simulink model "powersystem"  (R2024a)
settings: Solver=VariableStepAuto  StartTime=0.0  StopTime=10.0  RelTol=1e-3
libraries: spsThreePhaseVIMeasurementLib x6, spsThreePhaseBreakerLib x6, spsThreePhaseTransformerTwoWindingsLib x5, spsRMSLib x4, spsThreePhaseSourceLib x3, spsThreePhaseParallelRLCBranchLib x2, sps_lib x1
settings Model: Creator=acer  LastModifiedBy=acer

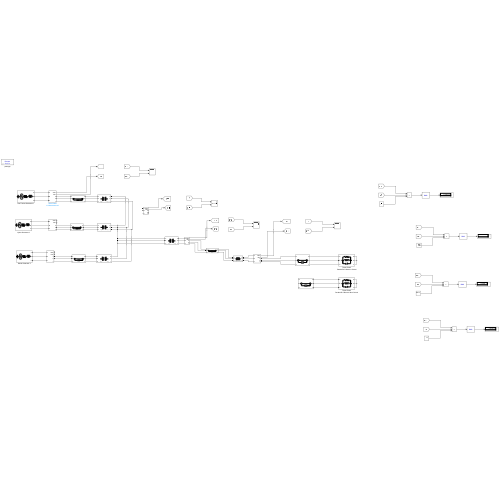
[thumbnail: Simulink's stored preview of the top-level diagram]
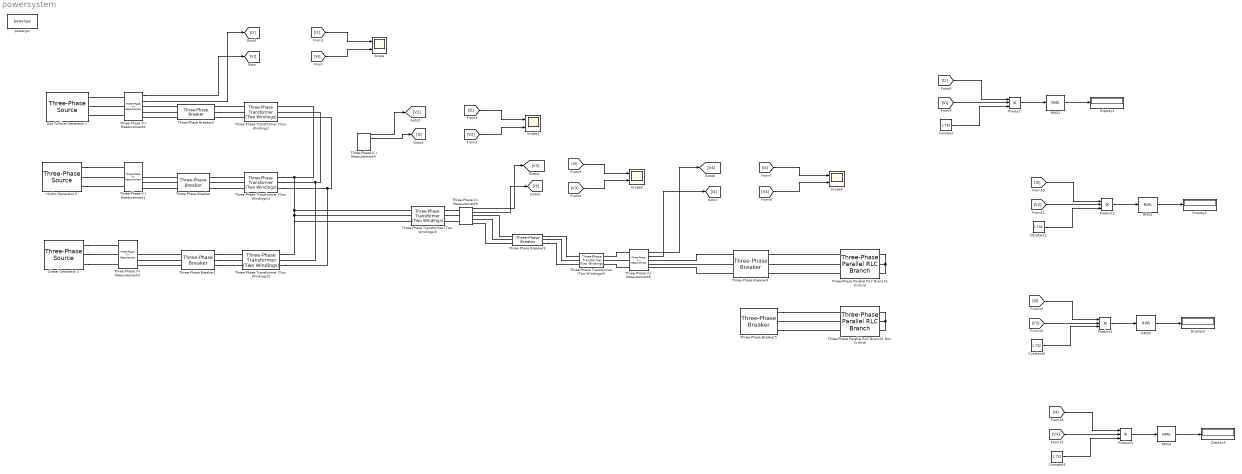
== system powersystem ==
  Constant{,1..3} (4 alike) : Constant  Value=1.732
  Diesel Genarator 3 : spsThreePhaseSourceLib/Three-Phase Source  InternalConnection=Yg  VoltagePhases=off  Voltage=10e3  PhaseAngle=0  Voltage_phases=[25e3 25e3 25e3]/sqrt(3)  PhaseAngles_phases=[0 -120 +120]  Frequency=50  NonIdealSource=on  SpecifyImpedance=off  Resistance=0.8  Inductance=16.58e-3  ShortCircuitLevel=100e6  BaseVoltage=11e3  XRratio=7  BusType=PV  Pref=400e4  Qref=0  Prefabc=[10e3, 10e3, 10e3]  Qrefabc=[0, 0, 0]  Qmin=-inf  Qmax=inf
  Display{1..4} (4 alike) : Display
  Gas Turbine Genarator 1 : spsThreePhaseSourceLib/Three-Phase Source  InternalConnection=Yg  VoltagePhases=off  Voltage=7e3  PhaseAngle=0  Voltage_phases=[25e3 25e3 25e3]/sqrt(3)  PhaseAngles_phases=[0 -120 +120]  Frequency=50  NonIdealSource=on  SpecifyImpedance=off  Resistance=0.8  Inductance=16.58e-3  ShortCircuitLevel=100e6  BaseVoltage=11e3  XRratio=7  BusType=PV  Pref=100e4  Qref=0  Prefabc=[10e3, 10e3, 10e3]  Qrefabc=[0, 0, 0]  Qmin=-inf  Qmax=inf
  Hydro Genarator 2 : spsThreePhaseSourceLib/Three-Phase Source  InternalConnection=Yg  VoltagePhases=off  Voltage=12e3  PhaseAngle=0  Voltage_phases=[25e3 25e3 25e3]/sqrt(3)  PhaseAngles_phases=[0 -120 +120]  Frequency=50  NonIdealSource=on  SpecifyImpedance=off  Resistance=0.8  Inductance=16.58e-3  ShortCircuitLevel=100e6  BaseVoltage=11e3  XRratio=7  BusType=PV  Pref=200e4  Qref=0  Prefabc=[10e3, 10e3, 10e3]  Qrefabc=[0, 0, 0]  Qmin=-inf  Qmax=inf
  Product{,1..3} (4 alike) : Product  Inputs=3
  RMS{1..4} (4 alike) : spsRMSLib/RMS  TrueRMS=on  Freq=60  RMSInit=120  Ts=0
  Scope{,1..3} (4 alike) : Scope  NumInputPorts=2
  Three-Phase Parallel RLC Branch1 Critical : spsThreePhaseParallelRLCBranchLib/Three-Phase Parallel RLC Branch  LConnTagsString=A|B|C  RConnTagsString=A|B|C  BranchType=RLC  Resistance=0.2  Inductance=0.489  Capacitance=0  Measurements=None
  Three-Phase Parallel RLC Branch1 Non Critical : spsThreePhaseParallelRLCBranchLib/Three-Phase Parallel RLC Branch  LConnTagsString=A|B|C  RConnTagsString=A|B|C  BranchType=RLC  Resistance=0.0682  Inductance=0.489  Capacitance=0  Measurements=None
  Three-Phase Transformer (Two Windings) : spsThreePhaseTransformerTwoWindingsLib/Three-Phase Transformer (Two Windings)  Winding1Connection=Yg  Winding2Connection=Yg  CoreType=Three single-phase transformers  SetSaturation=off  Hysteresis=off  DataFile='hysteresis'  SetInitialFlux=off  Measurements=Winding voltages  UNITS=SI  NominalPower=[ 1.5e6 , 50 ]  Winding1=[1.1e+04 0.3485 0.0215]  Winding2=[1.32e+05 0.002 0.000107]  Rm=1.0804e+06  Lm=3439.2  L0=0.5  Saturation=[0 0;0.66653 2292.3;277.72 2903.6]  InitialFluxes=[ 0.8 , -0.8 , 0.7 ]  BreakLoop=off  DiscreteSolver=Trapezoidal iterative  DataType=on  TransfoNumber=1
  Three-Phase Transformer (Two Windings)1 : spsThreePhaseTransformerTwoWindingsLib/Three-Phase Transformer (Two Windings)  Winding1Connection=Yg  Winding2Connection=Yg  CoreType=Three single-phase transformers  SetSaturation=off  Hysteresis=off  DataFile='hysteresis'  SetInitialFlux=off  Measurements=Winding voltages  UNITS=SI  NominalPower=[ 2.5e6 , 50 ]  Winding1=[1.2e+04 4.3218 0.55027]  Winding2=[1.32e+05 0.7938 0.10107]  Rm=1.0804e+06  Lm=3439.2  L0=0.5  Saturation=[0 0;0.66653 2292.3;277.72 2903.6]  InitialFluxes=[ 0.8 , -0.8 , 0.7 ]  BreakLoop=off  DiscreteSolver=Trapezoidal iterative  DataType=on  TransfoNumber=1
  Three-Phase Transformer (Two Windings)2 : spsThreePhaseTransformerTwoWindingsLib/Three-Phase Transformer (Two Windings)  Winding1Connection=Yg  Winding2Connection=Yg  CoreType=Three single-phase transformers  SetSaturation=off  Hysteresis=off  DataFile='hysteresis'  SetInitialFlux=off  Measurements=Winding voltages  UNITS=SI  NominalPower=[ 250e6 , 50 ]  Winding1=[1.0e+04 4.3218 0.55027]  Winding2=[1.32e+05 0.7938 0.10107]  Rm=1.0804e+06  Lm=3439.2  L0=0.5  Saturation=[0 0;0.66653 2292.3;277.72 2903.6]  InitialFluxes=[ 0.8 , -0.8 , 0.7 ]  BreakLoop=off  DiscreteSolver=Trapezoidal iterative  DataType=on  TransfoNumber=1
  Three-Phase Transformer (Two Windings)3 : spsThreePhaseTransformerTwoWindingsLib/Three-Phase Transformer (Two Windings)  Winding1Connection=Yg  Winding2Connection=Yg  CoreType=Three single-phase transformers  SetSaturation=off  Hysteresis=off  DataFile='hysteresis'  SetInitialFlux=off  Measurements=Winding voltages  UNITS=SI  NominalPower=[ 250e6 , 50 ]  Winding1=[1.32e+05 0.3218 0.55027]  Winding2=[1.1e+04 04.7938 0.010107]  Rm=1.0804e+06  Lm=3439.2  L0=0.5  Saturation=[0 0;0.66653 2292.3;277.72 2903.6]  InitialFluxes=[ 0.8 , -0.8 , 0.7 ]  BreakLoop=off  DiscreteSolver=Trapezoidal iterative  DataType=on  TransfoNumber=1
  Three-Phase Transformer (Two Windings)4 : spsThreePhaseTransformerTwoWindingsLib/Three-Phase Transformer (Two Windings)  Winding1Connection=Yg  Winding2Connection=Yg  CoreType=Three single-phase transformers  SetSaturation=off  Hysteresis=off  DataFile='hysteresis'  SetInitialFlux=off  Measurements=Winding voltages  UNITS=SI  NominalPower=[ 2.5e6 , 50 ]  Winding1=[1.1e+04 4.3218 0.55027]  Winding2=[0.4e+03 0.7938 0.10107]  Rm=1.0804e+06  Lm=3439.2  L0=0.5  Saturation=[0 0;0.66653 2292.3;277.72 2903.6]  InitialFluxes=[ 0.8 , -0.8 , 0.7 ]  BreakLoop=off  DiscreteSolver=Trapezoidal iterative  DataType=on  TransfoNumber=1
  Three-Phase V-I Measurement{1..6} (6 alike) : spsThreePhaseVIMeasurementLib/Three-Phase V-I Measurement  VoltageMeasurement=phase-to-phase  SetLabelV=off  LabelV=Vabc  Vpu=off  VpuLL=off  CurrentMeasurement=yes  SetLabelI=off  LabelI=Iabc  Ipu=off  Pbase=100e6  Vbase=500e3  OutputType=Complex  PhasorSimulation=off  PSBequivalent=0
  Three-Phase Breaker{,1..5} (6 alike) : spsThreePhaseBreakerLib/Three-Phase Breaker  InitialState=closed  SwitchA=on  SwitchB=on  SwitchC=on  SwitchTimes="[1/60  5/60]"  External=off  BreakerResistance=0.01  SnubberResistance=1e6  SnubberCapacitance=inf  Measurements=None
  powergui : sps_lib/powergui  Priority=1  SimulationMode=Discrete  SampleTime=50e-6  frequency=60  Iterations=50  frequencyindice=0  Pbase=100e6  ErrMax=1e-4  UnitsV=kV  UnitsW=MW  buscounter=0  FunctionMessages=off  echomessages=off  EnableUseOfTLC=off  CurrentSourceSwitches=off  DisableSnubberDevices=off  DisableRonSwitches=off  DisableVfSwitches=off  DisplayEquations=off  AutomaticDiscreteSolvers=off  SolverType=Tustin/Backward Euler (TBE)  Interpol=off  ExternalGateDelay=off  methode=off  Ts=100  x0status=blocks  SPID=on  SwTol=0  HookPort=off  NonlinearTolerance=1e-4  nMaxIteration=100  ContinueOnMaxIteration=off  RestoreLinks=warning  ResistiveCurrentMeasurement=off  Frange=[0:2:500]  Ylog=off  Xlog=on  ShowGrid=off  save=off  variable=ZData  structure=0  ZoomFFT=off  StartTime=0.0  cycles=1  DisplayStyle=1  fundamental=60  FreqAxis=off  MaxFrequency=1000  frequencyindicesteady=1  RmsSteady=1  display=off
  wires:
  Three-Phase V-I Measurement2/2 -> [I1]
  Three-Phase V-I Measurement2/1 -> [VI]
  [I1] -> Scope/1
  [VI] -> Scope/2
  [I2] -> Scope1/1
  [V2] -> Scope1/2
  Three-Phase V-I Measurement4/2 -> [I2]
  Three-Phase V-I Measurement4/1 -> [V2]
  Three-Phase V-I Measurement5/1 -> [V3]
  [V3] -> Scope2/2
  [I3] -> Scope2/1
  Three-Phase V-I Measurement5/2 -> [I3]
  [V4] -> Scope3/2
  [I4] -> Scope3/1
  Three-Phase V-I Measurement6/1 -> [V4]
  Three-Phase V-I Measurement6/2 -> [I4]
  RMS1/1 -> Display1/1
  Constant/1 -> Product/3
  Product/1 -> RMS1/1
  [I1] -> Product/1
  [VI] -> Product/2
  RMS2/1 -> Display2/1
  Constant1/1 -> Product1/3
  Product1/1 -> RMS2/1
  [I2] -> Product1/1
  [V2] -> Product1/2
  [I3] -> Product2/1
  Product2/1 -> RMS3/1
  RMS3/1 -> Display3/1
  Constant2/1 -> Product2/3
  [V3] -> Product2/2
  [I4] -> Product3/1
  Product3/1 -> RMS4/1
  RMS4/1 -> Display4/1
  Constant3/1 -> Product3/3
  [V4] -> Product3/2
  connections:
  Gas Turbine Genarator 1/RConn1 -- Three-Phase V-I Measurement2/LConn1
  Gas Turbine Genarator 1/RConn2 -- Three-Phase V-I Measurement2/LConn2
  Gas Turbine Genarator 1/RConn3 -- Three-Phase V-I Measurement2/LConn3
  Hydro Genarator 2/RConn1 -- Three-Phase V-I Measurement1/LConn1
  Hydro Genarator 2/RConn2 -- Three-Phase V-I Measurement1/LConn2
  Hydro Genarator 2/RConn3 -- Three-Phase V-I Measurement1/LConn3
  Diesel Genarator 3/RConn1 -- Three-Phase V-I Measurement3/LConn1
  Diesel Genarator 3/RConn2 -- Three-Phase V-I Measurement3/LConn2
  Diesel Genarator 3/RConn3 -- Three-Phase V-I Measurement3/LConn3
  Three-Phase Transformer (Two Windings)1/RConn1 -- Three-Phase Transformer (Two Windings)3/LConn1 -- Three-Phase Transformer (Two Windings)3/LConn2 -- Three-Phase Transformer (Two Windings)3/LConn3 -- Three-Phase Transformer (Two Windings)2/RConn1 -- Three-Phase Transformer (Two Windings)/RConn1
  Three-Phase Transformer (Two Windings)1/RConn2 -- Three-Phase Transformer (Two Windings)2/RConn2 -- Three-Phase Transformer (Two Windings)/RConn2
  Three-Phase Transformer (Two Windings)1/RConn3 -- Three-Phase Transformer (Two Windings)2/RConn3 -- Three-Phase Transformer (Two Windings)/RConn3
  Three-Phase Breaker1/LConn1 -- Three-Phase V-I Measurement3/RConn1
  Three-Phase Breaker1/LConn2 -- Three-Phase V-I Measurement3/RConn2
  Three-Phase Breaker1/LConn3 -- Three-Phase V-I Measurement3/RConn3
  Three-Phase Breaker1/RConn3 -- Three-Phase Transformer (Two Windings)2/LConn3
  Three-Phase Breaker1/RConn2 -- Three-Phase Transformer (Two Windings)2/LConn2
  Three-Phase Breaker1/RConn1 -- Three-Phase Transformer (Two Windings)2/LConn1
  Three-Phase Breaker/LConn3 -- Three-Phase V-I Measurement1/RConn3
  Three-Phase Breaker/LConn2 -- Three-Phase V-I Measurement1/RConn2
  Three-Phase Breaker/LConn1 -- Three-Phase V-I Measurement1/RConn1
  Three-Phase Breaker/RConn3 -- Three-Phase Transformer (Two Windings)1/LConn3
  Three-Phase Breaker/RConn2 -- Three-Phase Transformer (Two Windings)1/LConn2
  Three-Phase Breaker/RConn1 -- Three-Phase Transformer (Two Windings)1/LConn1
  Three-Phase Breaker2/LConn3 -- Three-Phase V-I Measurement2/RConn3
  Three-Phase Breaker2/LConn2 -- Three-Phase V-I Measurement2/RConn2
  Three-Phase Breaker2/LConn1 -- Three-Phase V-I Measurement2/RConn1
  Three-Phase Breaker2/RConn1 -- Three-Phase Transformer (Two Windings)/LConn1
  Three-Phase Breaker2/RConn2 -- Three-Phase Transformer (Two Windings)/LConn2
  Three-Phase Breaker2/RConn3 -- Three-Phase Transformer (Two Windings)/LConn3
  Three-Phase V-I Measurement5/LConn3 -- Three-Phase Transformer (Two Windings)3/RConn3
  Three-Phase V-I Measurement5/LConn2 -- Three-Phase Transformer (Two Windings)3/RConn2
  Three-Phase V-I Measurement5/LConn1 -- Three-Phase Transformer (Two Windings)3/RConn1
  Three-Phase Parallel RLC Branch1 Critical/RConn2 -- Three-Phase Parallel RLC Branch1 Critical/RConn3 -- Three-Phase Parallel RLC Branch1 Critical/RConn1
  Three-Phase V-I Measurement6/LConn1 -- Three-Phase Transformer (Two Windings)4/RConn1
  Three-Phase V-I Measurement6/LConn3 -- Three-Phase Transformer (Two Windings)4/RConn3
  Three-Phase V-I Measurement6/LConn2 -- Three-Phase Transformer (Two Windings)4/RConn2
  Three-Phase Parallel RLC Branch1 Non Critical/RConn2 -- Three-Phase Parallel RLC Branch1 Non Critical/RConn3 -- Three-Phase Parallel RLC Branch1 Non Critical/RConn1
  Three-Phase Breaker3/RConn3 -- Three-Phase Transformer (Two Windings)4/LConn3
  Three-Phase Breaker3/RConn2 -- Three-Phase Transformer (Two Windings)4/LConn2
  Three-Phase Breaker3/RConn1 -- Three-Phase Transformer (Two Windings)4/LConn1
  Three-Phase Breaker3/LConn3 -- Three-Phase V-I Measurement5/RConn3
  Three-Phase Breaker3/LConn2 -- Three-Phase V-I Measurement5/RConn2
  Three-Phase Breaker3/LConn1 -- Three-Phase V-I Measurement5/RConn1
  Three-Phase Breaker4/LConn3 -- Three-Phase V-I Measurement6/RConn3
  Three-Phase Breaker4/LConn2 -- Three-Phase V-I Measurement6/RConn2
  Three-Phase Breaker4/LConn1 -- Three-Phase V-I Measurement6/RConn1
  Three-Phase Breaker4/RConn1 -- Three-Phase Parallel RLC Branch1 Critical/LConn1
  Three-Phase Breaker4/RConn2 -- Three-Phase Parallel RLC Branch1 Critical/LConn2
  Three-Phase Breaker4/RConn3 -- Three-Phase Parallel RLC Branch1 Critical/LConn3
  Three-Phase Breaker5/RConn1 -- Three-Phase Parallel RLC Branch1 Non Critical/LConn1
  Three-Phase Breaker5/RConn2 -- Three-Phase Parallel RLC Branch1 Non Critical/LConn2
  Three-Phase Breaker5/RConn3 -- Three-Phase Parallel RLC Branch1 Non Critical/LConn3
